simulink model "rocket_simulator"  (R2024b)
settings: Solver=ode45  StartTime=0.0  StopTime=200  RelTol=1e-5  AbsTol=1e-7
undefined symbols (not defined in the file or in its folder): ENG, MSL
libraries: engine_library x1, rocketdynamics_library x1
settings Model: Creator=Leonardo Perina  LastModifiedBy=Leonardo Perina

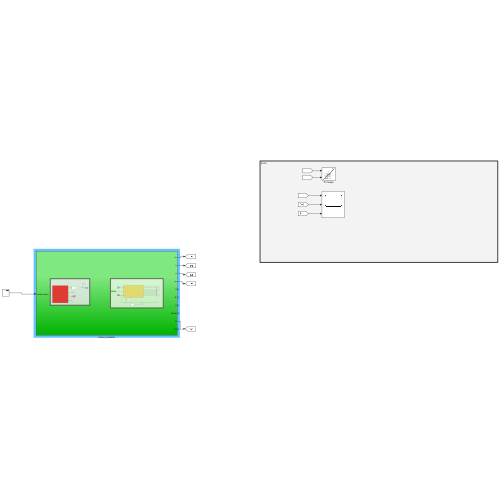
[thumbnail: Simulink's stored preview of the top-level diagram]
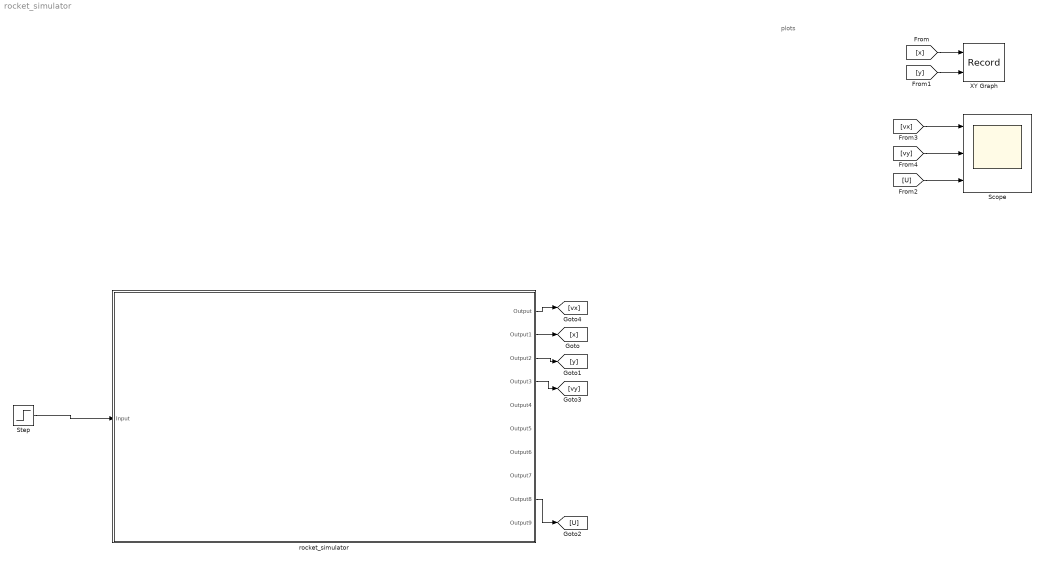
== system rocket_simulator ==
  note: plots
  Scope : Scope  NumInputPorts=3
  Step : Step  SampleTime=0
  XY Graph : Record  FileSettingsInternal="{\"entries\":[{\"content\":{\"excelSettings\":{\"content\":{},\"type\":\"Streamout.ExcelSettings\"}},\"type\":\"Streamout.FileSettingStorage\",\"uuid\":\"\"}],\"packageUris\":[\"http:\\/\\/schema.mathworks.com\\/mf0\\/streamout_blocks\\/R2020a\"],\"version\":\"1.0\"}"  Layout=[1 1]  SignalsInternal="{\"entries\":[{\"content\":{\"signals\":[{\"content\":{\"blockPath\":[],\"dimensions\":[1,1],\"domain\":\"\",\"lineColor\":\"#a2142f\",\"plots\":[ 1 ],\"port\":1,\"sid\":[\"\"],\"signalID\":1,\"signalName\":\"From\"},\"type\":\"RecordBlkView.Signal\",\"uuid\":\"\"},{\"content\":{\"blockPath\":[],\"dimensions\":[1,1],\"domain\":\"\",\"lineColor\":\"#139fff\",\"plots\":[ 1 ],\"port\":2,\"sid\":[\"\"],\"signalID\":2,\"signalName\":\"From1\"},\"type\":\"RecordBlkView.Signal\",\"uuid\":\"\"}]},\"type\":\"RecordBlkView.InputSignals\",\"uuid\":\"\"}],\"packageUris\":[\"http:\\/\\/schema.mathworks.com\\/mf0\\/streamout_blocks\\/R2020a\"],\"version\":\"1.0\"}"  VisualizationBindings="{\"xyplotplugin\":{\"info\":[{\"series\":[{\"bindingParametersList\":[{\"parameter\":\"X-Axis\",\"signalID\":1,\"signalName\":\"From\"},{\"parameter\":\"Y-Axis\",\"signalID\":2,\"signalName\":\"From1\"}],\"seriesID\":0}],\"subplotID\":1}]}}"  CompatibilityTag=XY
  rocket_simulator : Subsystem
  wires:
  rocket_simulator/2(Output1) -> [x]
  [x] -> XY Graph/1
  rocket_simulator/3(Output2) -> [y]
  [y] -> XY Graph/2
  Step/1 -> rocket_simulator/1(Input)
  rocket_simulator/9(Output8) -> [U]
  rocket_simulator/4(Output3) -> [vy]
  rocket_simulator/1(Output) -> [vx]
  [vx] -> Scope/1
  [vy] -> Scope/2
  [U] -> Scope/3

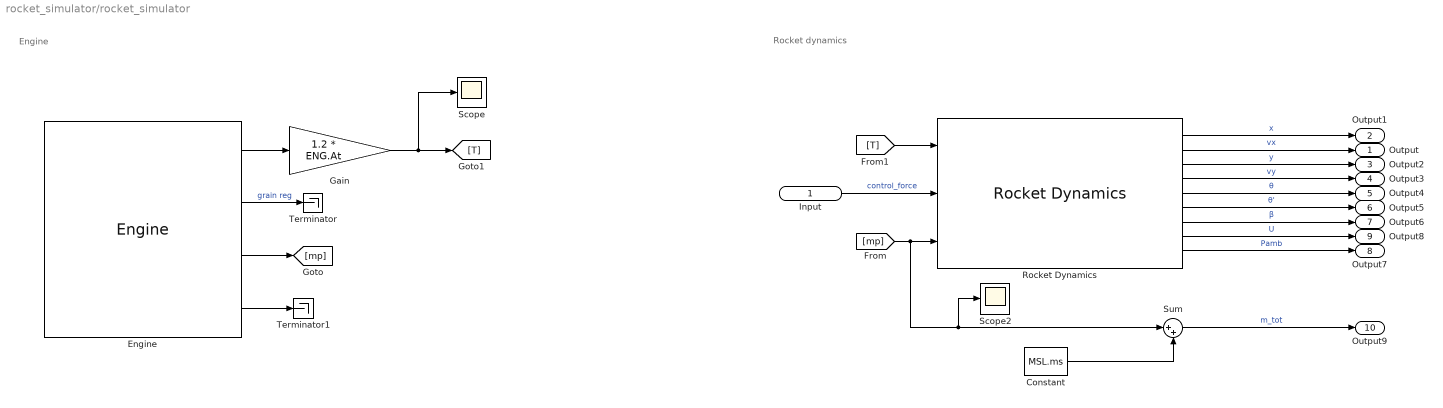
== system rocket_simulator/rocket_simulator ==
  note: Rocket dynamics
  note: Engine
  Input : Inport
  Constant : Constant  Value=MSL.ms
  Engine : engine_library/Engine  SystemSampleTime=-1  VariantActivationTime=update diagram  AllowFlexibleInterface=on  Latency=0  AutoFrameSizeCalculation=off
  Gain : Gain  Gain=1.2 * ENG.At
  Rocket Dynamics : rocketdynamics_library/Rocket Dynamics  SystemSampleTime=-1  VariantActivationTime=update diagram  AllowFlexibleInterface=on  Latency=0  AutoFrameSizeCalculation=off
  Scope : Scope
  Scope2 : Scope
  Sum : Sum  Inputs=|++
  Terminator : Terminator
  Terminator1 : Terminator
  Output : Outport
  Output1 : Outport  Port=2
  Output2 : Outport  Port=3
  Output3 : Outport  Port=4
  Output4 : Outport  Port=5
  Output5 : Outport  Port=6
  Output6 : Outport  Port=7
  Output7 : Outport  Port=8
  Output8 : Outport  Port=9
  Output9 : Outport  Port=10
  wires:
  Gain/1 -> Scope/1, [T]
  Engine/4 -> Terminator1/1
  Engine/3 -> [mp]
  Rocket Dynamics/8 -> Output8/1  "U"
  [T] -> Rocket Dynamics/1
  [mp] -> Scope2/1, Sum/1, Rocket Dynamics/3
  Engine/2 -> Terminator/1  "grain reg"
  Engine/1 -> Gain/1
  Input/1 -> Rocket Dynamics/2  "control_force"
  Rocket Dynamics/2 -> Output/1  "vx"
  Rocket Dynamics/1 -> Output1/1  "x"
  Rocket Dynamics/3 -> Output2/1  "y"
  Rocket Dynamics/4 -> Output3/1  "vy"
  Rocket Dynamics/5 -> Output4/1  "θ"
  Rocket Dynamics/6 -> Output5/1  "θ'"
  Rocket Dynamics/7 -> Output6/1  "β"
  Rocket Dynamics/9 -> Output7/1  "Pamb"
  Sum/1 -> Output9/1  "m_tot"
  Constant/1 -> Sum/2
